simulink model "Aufgabe_7_3_ref"  (R2021b)
settings: Solver=VariableStepAuto  StartTime=0.0  StopTime=10.0  RelTol=1e-3
libraries: simulink x9, simulink_extras x3
settings Model: Creator=weixiong  LastModifiedBy=weixiong

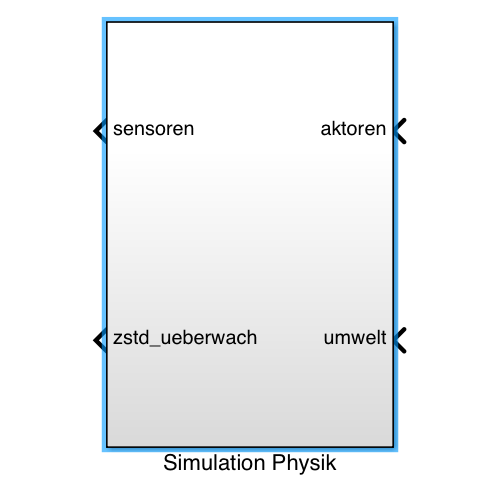
[thumbnail: Simulink's stored preview of the top-level diagram]
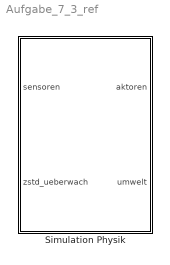
== system Aufgabe_7_3_ref ==
  Simulation Physik : Subsystem

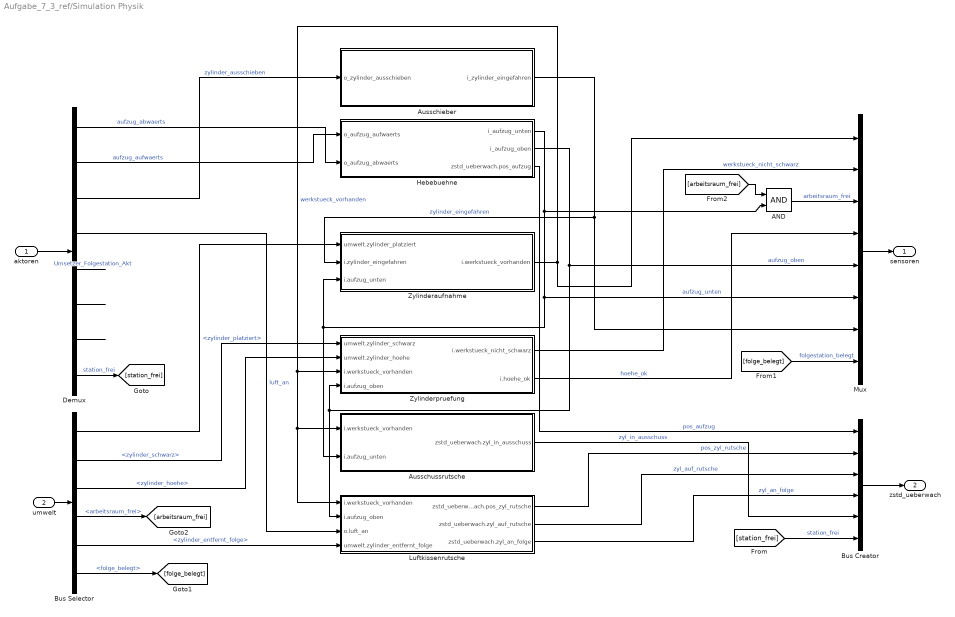
== system Aufgabe_7_3_ref/Simulation Physik ==
  aktoren : Inport
  umwelt : Inport  Port=2
  AND : Logic  AllPortsSameDT=off  OutDataTypeStr=boolean
  Ausschieber : Subsystem
  Ausschussrutsche : Subsystem
  Bus Creator : BusCreator  Inputs=6
  Bus Selector : BusSelector  OutputSignals=zylinder_platziert,zylinder_schwarz,zylinder_hoehe,arbeitsraum_frei,zylinder_entfernt_folge,folge_belegt
  Demux : Demux  Outputs=8
  Hebebuehne : Subsystem
  Luftkissenrutsche : Subsystem
  Mux : Mux  Inputs=8
  Zylinderaufnahme : Subsystem
  Zylinderpruefung : Subsystem
  sensoren : Outport  VectorParamsAs1DForOutWhenUnconnected=off
  zstd_ueberwach : Outport  Port=2  VectorParamsAs1DForOutWhenUnconnected=off
  wires:
  Bus Selector/5 -> Luftkissenrutsche/4(umwelt.zylinder_entfernt_folge)  "<zylinder_entfernt_folge>"
  Bus Selector/6 -> [folge_belegt]  "<folge_belegt>"
  Hebebuehne/1(i_aufzug_unten) -> AND/2, Ausschussrutsche/2(i.aufzug_unten), Zylinderaufnahme/3(i.aufzug_unten), Mux/6  "aufzug_unten"
  Ausschieber/1(i_zylinder_eingefahren) -> Mux/7, Zylinderaufnahme/2(i.zylinder_eingefahren)  "zylinder_eingefahren"
  [folge_belegt] -> Mux/8  "folgestation_belegt"
  Demux/2 -> Hebebuehne/1(o_aufzug_aufwaerts)  "aufzug_aufwaerts"
  umwelt/1 -> Bus Selector/1
  Luftkissenrutsche/2(zstd_ueberwach.zyl_auf_rutsche) -> Bus Creator/3  "zyl_auf_rutsche"
  aktoren/1 -> Demux/1
  Mux/1 -> sensoren/1
  AND/1 -> Mux/3  "arbeitsraum_frei"
  Demux/1 -> Hebebuehne/2(o_aufzug_abwaerts)  "aufzug_abwaerts"
  Hebebuehne/2(i_aufzug_oben) -> Luftkissenrutsche/2(i.aufzug_oben), Zylinderpruefung/4(i.aufzug_oben), Mux/5  "aufzug_oben"
  Demux/4 -> Luftkissenrutsche/3(o.luft_an)  "luft_an"
  [arbeitsraum_frei] -> AND/1
  Zylinderaufnahme/1(i.werkstueck_vorhanden) -> Mux/1, Luftkissenrutsche/1(i.werkstueck_vorhanden), Ausschussrutsche/1(i.werkstueck_vorhanden), Zylinderpruefung/3(i.werkstueck_vorhanden)  "werkstueck_vorhanden"
  Bus Creator/1 -> zstd_ueberwach/1
  Bus Selector/2 -> Zylinderpruefung/1(umwelt.zylinder_schwarz)  "<zylinder_schwarz>"
  Luftkissenrutsche/3(zstd_ueberwach.zyl_an_folge) -> Bus Creator/4  "zyl_an_folge"
  Zylinderpruefung/1(i.werkstueck_nicht_schwarz) -> Mux/2  "werkstueck_nicht_schwarz"
  Demux/8 -> [station_frei]  "station_frei"
  Bus Selector/4 -> [arbeitsraum_frei]  "<arbeitsraum_frei>"
  Bus Selector/1 -> Zylinderaufnahme/1(umwelt.zylinder_platziert)  "<zylinder_platziert>"
  Zylinderpruefung/2(i.hoehe_ok) -> Mux/4  "hoehe_ok"
  [station_frei] -> Bus Creator/6  "station_frei"
  Hebebuehne/3(zstd_ueberwach.pos_aufzug) -> Bus Creator/1  "pos_aufzug"
  Bus Selector/3 -> Zylinderpruefung/2(umwelt.zylinder_hoehe)  "<zylinder_hoehe>"
  Ausschussrutsche/1(zstd_ueberwach.zyl_in_ausschuss) -> Bus Creator/5  "zyl_in_ausschuss"
  Demux/3 -> Ausschieber/1(o_zylinder_ausschieben)  "zylinder_ausschieben"
  Luftkissenrutsche/1(zstd_ueberwach.pos_zyl_rutsche) -> Bus Creator/2  "pos_zyl_rutsche"
  Demux/5 -> ?  "Umsetzer_Folgestation_Akt"
  Demux/6 -> ?
  Demux/7 -> ?

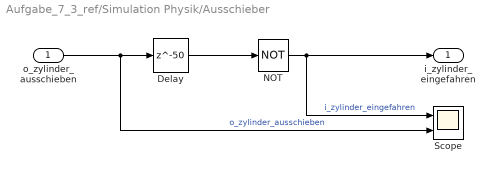
== system Aufgabe_7_3_ref/Simulation Physik/Ausschieber ==
  o_zylinder_ausschieben : Inport
  Delay : Delay  DelayLength=50
  NOT : Logic  Operator=NOT  AllPortsSameDT=off  OutDataTypeStr=boolean
  Scope : Scope  NumInputPorts=2
  i_zylinder_eingefahren : Outport
  wires:
  o_zylinder_ausschieben/1 -> Scope/2, Delay/1  "o_zylinder_ausschieben"
  Delay/1 -> NOT/1
  NOT/1 -> Scope/1, i_zylinder_eingefahren/1  "i_zylinder_eingefahren"

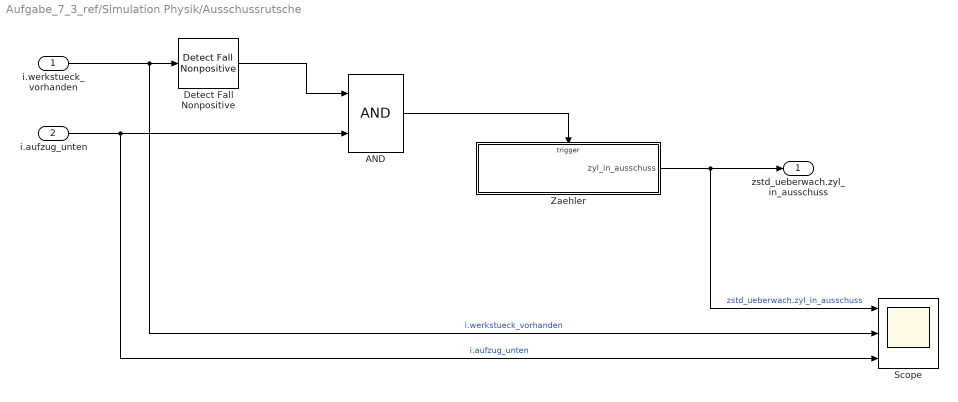
== system Aufgabe_7_3_ref/Simulation Physik/Ausschussrutsche ==
  i.werkstueck_vorhanden : Inport
  i.aufzug_unten : Inport  Port=2
  AND : Logic  AllPortsSameDT=off  OutDataTypeStr=boolean
  Detect Fall Nonpositive : simulink/Logic and Bit Operations/Detect Fall Nonpositive  vinit=0  OutDataTypeStr=boolean
      settings: SourceProductBaseCode=SL
  Scope : Scope  NumInputPorts=3
  Zaehler : Subsystem  TreatAsAtomicUnit=on
  zstd_ueberwach.zyl_in_ausschuss : Outport
  wires:
  i.werkstueck_vorhanden/1 -> Scope/2, Detect Fall Nonpositive/1  "i.werkstueck_vorhanden"
  Detect Fall Nonpositive/1 -> AND/1
  i.aufzug_unten/1 -> Scope/3, AND/2  "i.aufzug_unten"
  AND/1 -> Zaehler/Trigger
  Zaehler/1(zyl_in_ausschuss) -> Scope/1, zstd_ueberwach.zyl_in_ausschuss/1  "zstd_ueberwach.zyl_in_ausschuss"

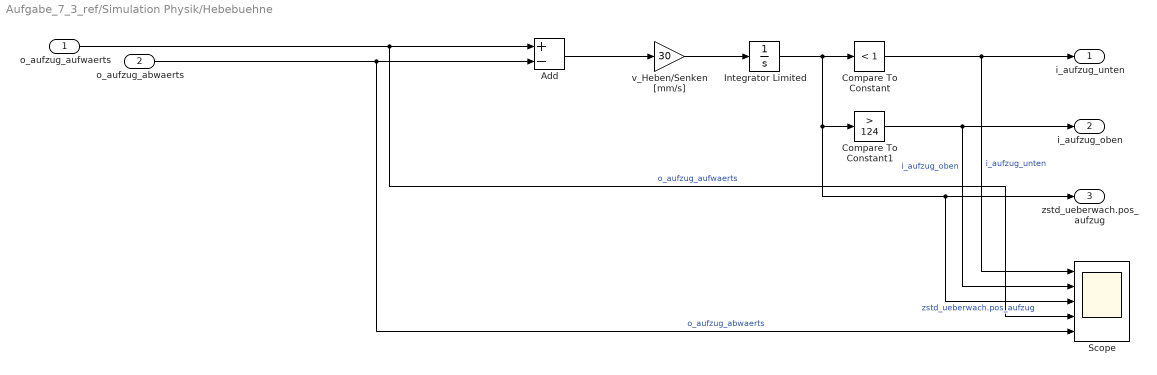
== system Aufgabe_7_3_ref/Simulation Physik/Hebebuehne ==
  o_aufzug_aufwaerts : Inport
  o_aufzug_abwaerts : Inport  Port=2
  Add : Sum  Inputs=+-
  Compare To Constant : simulink/Logic and Bit Operations/Compare To Constant  relop=<  const=1  OutDataTypeStr=boolean
  Compare To Constant1 : simulink/Logic and Bit Operations/Compare To Constant  relop=>  const=124  OutDataTypeStr=boolean
  Integrator Limited : Integrator  LimitOutput=on  UpperSaturationLimit=125  LowerSaturationLimit=0
  Scope : Scope  NumInputPorts=5
  v_Heben/Senken [mm/s] : Gain  Gain=30
  i_aufzug_unten : Outport
  i_aufzug_oben : Outport  Port=2
  zstd_ueberwach.pos_aufzug : Outport  Port=3
  wires:
  v_Heben/Senken [mm/s]/1 -> Integrator Limited/1
  o_aufzug_aufwaerts/1 -> Add/1, Scope/4  "o_aufzug_aufwaerts"
  o_aufzug_abwaerts/1 -> Scope/5, Add/2  "o_aufzug_abwaerts"
  Add/1 -> v_Heben/Senken [mm/s]/1
  Integrator Limited/1 -> Scope/3, zstd_ueberwach.pos_aufzug/1, Compare To Constant1/1, Compare To Constant/1  "zstd_ueberwach.pos_aufzug"
  Compare To Constant/1 -> i_aufzug_unten/1, Scope/1  "i_aufzug_unten"
  Compare To Constant1/1 -> i_aufzug_oben/1, Scope/2  "i_aufzug_oben"

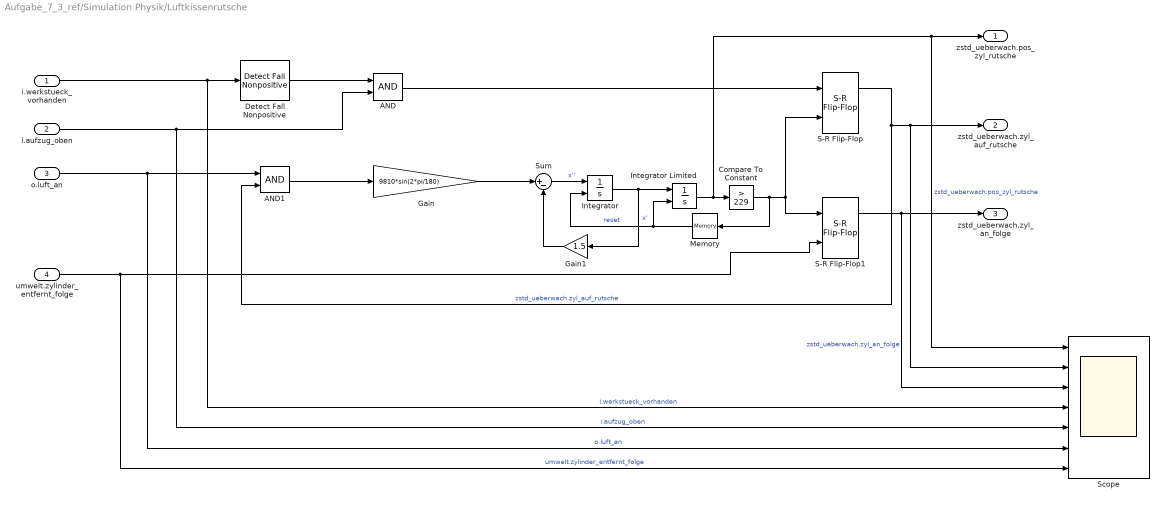
== system Aufgabe_7_3_ref/Simulation Physik/Luftkissenrutsche ==
  i.werkstueck_vorhanden : Inport
  i.aufzug_oben : Inport  Port=2
  o.luft_an : Inport  Port=3
  umwelt.zylinder_entfernt_folge : Inport  Port=4
  AND : Logic  AllPortsSameDT=off  OutDataTypeStr=boolean
  AND1 : Logic  AllPortsSameDT=off  OutDataTypeStr=boolean
  Compare To Constant : simulink/Logic and Bit Operations/Compare To Constant  relop=>  const=229  OutDataTypeStr=boolean
  Detect Fall Nonpositive : simulink/Logic and Bit Operations/Detect Fall Nonpositive  vinit=0  OutDataTypeStr=boolean
      settings: SourceProductBaseCode=SL
  Gain : Gain  Gain=9810*sin(2*pi/180)
  Gain1 : Gain  Gain=1.5
  Integrator : Integrator  ExternalReset=rising
  Integrator Limited : Integrator  ExternalReset=rising  LimitOutput=on  UpperSaturationLimit=230  LowerSaturationLimit=0
  Memory : Memory
  S-R Flip-Flop : simulink_extras/Flip Flops/S-R Flip-Flop  initial_condition=0
  S-R Flip-Flop1 : simulink_extras/Flip Flops/S-R Flip-Flop  initial_condition=0
  Scope : Scope  NumInputPorts=7
  Sum : Sum  Inputs=|+-
  zstd_ueberwach.pos_zyl_rutsche : Outport
  zstd_ueberwach.zyl_auf_rutsche : Outport  Port=2
  zstd_ueberwach.zyl_an_folge : Outport  Port=3
  wires:
  i.aufzug_oben/1 -> Scope/5, AND/2  "i.aufzug_oben"
  i.werkstueck_vorhanden/1 -> Scope/4, Detect Fall Nonpositive/1  "i.werkstueck_vorhanden"
  Detect Fall Nonpositive/1 -> AND/1
  AND/1 -> S-R Flip-Flop/1
  o.luft_an/1 -> Scope/6, AND1/1  "o.luft_an"
  S-R Flip-Flop/1 -> AND1/2, zstd_ueberwach.zyl_auf_rutsche/1, Scope/2  "zstd_ueberwach.zyl_auf_rutsche"
  Compare To Constant/1 -> Memory/1, S-R Flip-Flop/2, S-R Flip-Flop1/1
  Gain1/1 -> Sum/2
  Gain/1 -> Sum/1
  Sum/1 -> Integrator/1  "x''"
  Integrator/1 -> Gain1/1, Integrator Limited/1  "x'"
  Integrator Limited/1 -> zstd_ueberwach.pos_zyl_rutsche/1, Scope/1, Compare To Constant/1  "zstd_ueberwach.pos_zyl_rutsche"
  S-R Flip-Flop1/1 -> Scope/3, zstd_ueberwach.zyl_an_folge/1  "zstd_ueberwach.zyl_an_folge"
  Memory/1 -> Integrator Limited/2, Integrator/2  "reset"
  AND1/1 -> Gain/1
  umwelt.zylinder_entfernt_folge/1 -> Scope/7, S-R Flip-Flop1/2  "umwelt.zylinder_entfernt_folge"

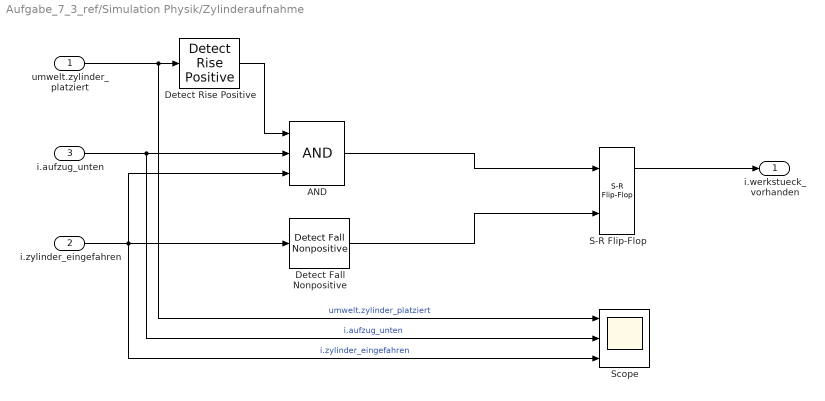
== system Aufgabe_7_3_ref/Simulation Physik/Zylinderaufnahme ==
  umwelt.zylinder_platziert : Inport
  i.zylinder_eingefahren : Inport  Port=2
  i.aufzug_unten : Inport  Port=3
  AND : Logic  Inputs=3  AllPortsSameDT=off  OutDataTypeStr=boolean
  Detect Fall Nonpositive : simulink/Logic and Bit Operations/Detect Fall Nonpositive  vinit=0  OutDataTypeStr=boolean
      settings: SourceProductBaseCode=SL
  Detect Rise Positive : simulink/Logic and Bit Operations/Detect Rise Positive  vinit=0  OutDataTypeStr=boolean
  S-R Flip-Flop : simulink_extras/Flip Flops/S-R Flip-Flop  initial_condition=0
  Scope : Scope  NumInputPorts=3
  i.werkstueck_vorhanden : Outport
  wires:
  Detect Rise Positive/1 -> AND/1
  umwelt.zylinder_platziert/1 -> Scope/1, Detect Rise Positive/1  "umwelt.zylinder_platziert"
  i.zylinder_eingefahren/1 -> Scope/3, Detect Fall Nonpositive/1, AND/3  "i.zylinder_eingefahren"
  i.aufzug_unten/1 -> Scope/2, AND/2  "i.aufzug_unten"
  AND/1 -> S-R Flip-Flop/1
  S-R Flip-Flop/1 -> i.werkstueck_vorhanden/1
  Detect Fall Nonpositive/1 -> S-R Flip-Flop/2

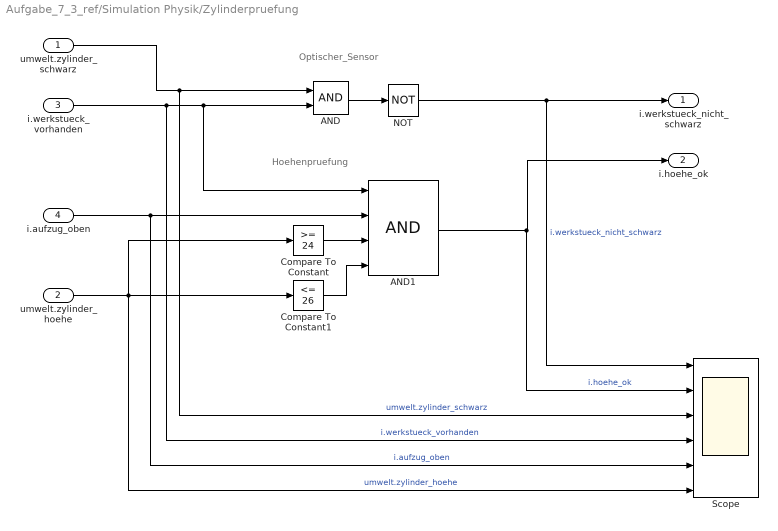
== system Aufgabe_7_3_ref/Simulation Physik/Zylinderpruefung ==
  note: Hoehenpruefung
  note: Optischer_Sensor
  umwelt.zylinder_schwarz : Inport
  umwelt.zylinder_hoehe : Inport  Port=2
  i.werkstueck_vorhanden : Inport  Port=3
  i.aufzug_oben : Inport  Port=4
  AND : Logic  AllPortsSameDT=off  OutDataTypeStr=boolean
  AND1 : Logic  Inputs=4  AllPortsSameDT=off  OutDataTypeStr=boolean
  Compare To Constant : simulink/Logic and Bit Operations/Compare To Constant  relop=>=  const=24  OutDataTypeStr=boolean
  Compare To Constant1 : simulink/Logic and Bit Operations/Compare To Constant  relop=<=  const=26  OutDataTypeStr=boolean
  NOT : Logic  Operator=NOT  AllPortsSameDT=off  OutDataTypeStr=boolean
  Scope : Scope  NumInputPorts=6
  i.werkstueck_nicht_schwarz : Outport
  i.hoehe_ok : Outport  Port=2
  wires:
  i.werkstueck_vorhanden/1 -> Scope/4, AND/2, AND1/1  "i.werkstueck_vorhanden"
  i.aufzug_oben/1 -> Scope/5, AND1/2  "i.aufzug_oben"
  umwelt.zylinder_schwarz/1 -> Scope/3, AND/1  "umwelt.zylinder_schwarz"
  AND/1 -> NOT/1
  NOT/1 -> Scope/1, i.werkstueck_nicht_schwarz/1  "i.werkstueck_nicht_schwarz"
  umwelt.zylinder_hoehe/1 -> Compare To Constant1/1, Scope/6, Compare To Constant/1  "umwelt.zylinder_hoehe"
  Compare To Constant/1 -> AND1/3
  Compare To Constant1/1 -> AND1/4
  AND1/1 -> Scope/2, i.hoehe_ok/1  "i.hoehe_ok"

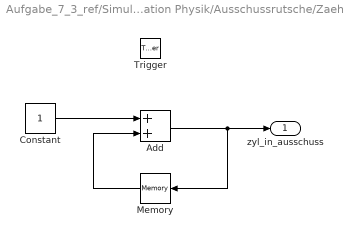
== system Aufgabe_7_3_ref/Simulation Physik/Ausschussrutsche/Zaehler ==
  Trigger : TriggerPort  VariantControl=Variant
  Add : Sum
  Constant : Constant
  Memory : Memory  InheritSampleTime=on
  zyl_in_ausschuss : Outport
  wires:
  Constant/1 -> Add/1
  Add/1 -> Memory/1, zyl_in_ausschuss/1
  Memory/1 -> Add/2
